simulink model "dynmodelinglinearmpc"  (R2019a)
settings: Solver=FixedStepAuto  StartTime=0.0  StopTime=25  RelTol=1e-3
model workspace (MAT data in the model file):
  op_trim1 : opcond.OperatingReport (value not decoded)
values from neighbouring files (symbols this model uses):
  k = convhulln(p)    [main.m]
undefined symbols (not defined in the file or in its folder): J, L, Mf, R, Rc, Rw
libraries: mpclib x1, mobileRoboticsLib x1
settings Model: Creator=Malicious  LastModifiedBy=colson
settings DataIOCC: ExternalInput=getinputstruct(op_trim1)  InitialState=getstatestruct(op_trim1)  LoadExternalInput=on  ReturnWorkspaceOutputs=off
settings DebuggingCC: PregeneratedLibrarySubsystemCodeDiagnostic=none  ArithmeticOperatorsInVariantConditions=warning
settings SFSimCC: SimUseLocalCustomCode=off
settings RTWCC: RTWUseLocalCustomCode=off

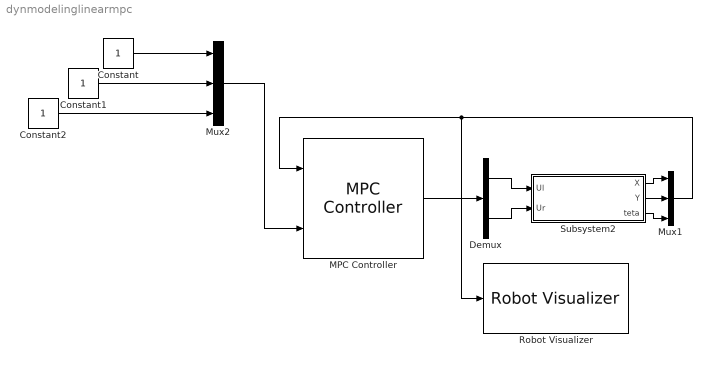
== system dynmodelinglinearmpc ==
  Constant : Constant
  Constant1 : Constant
  Constant2 : Constant
  Demux : Demux  Outputs=2
  MPC Controller : mpclib/MPC Controller  SCDEnableBlockLinearizationSpecification=on  mpcobj=mpc1  is_multiple=0  enable_value=0  return_u0=off  updateMPCinCallerWorkspace=on  md_inport=off  mv_inport=off  uref_inport=off  return_cost=off  return_mvseq=off  return_qpstatus=off  return_xseq=off  return_state=off  return_ovseq=off  state_inport=off  umin_inport=off  umax_inport=off  ymin_inport=off  ymax_inport=off  cc_inport=off  ywt_inport=off  uwt_inport=off  duwt_inport=off  rhoeps_inport=off  pm_inport=off  MaximumP=10  HorizonChoice=FixedHorizon  n_ts=0.1  n_p=10  n_mv=2  n_md=0  n_ud=0  n_mo=3  n_uo=0  BlockDataType=double  SampleTimeInherited=off  switch_inport=off
  Mux1 : Mux  Inputs=3
  Mux2 : Mux  Inputs=3
  Robot Visualizer : mobileRoboticsLib/Environments/Robot Visualizer  robotRadius=0.2  showTrajectory=on  hasWaypoints=off  hasLidar=off  sensorOffset=[ 0, 0 ]  scanAngles=[ -pi/4, 0, pi/4 ]  hasObjDetector=off  objDetectorOffset=[ 0, 0 ]  objDetectorAngle=0  objDetectorFOV=pi/4  objDetectorMaxRange=5  objectColors=[ 1, 0, 0; 0, 1, 0; 0, 0, 1 ]  objectMarkers=s
      settings: SourceProductName=Mobile Robotics Simulation Library
  Subsystem2 : Subsystem
  wires:
  MPC Controller/1 -> Demux/1
  Mux1/1 -> Robot Visualizer/1, MPC Controller/1
  Subsystem2/3(teta) -> Mux1/3
  Subsystem2/2(Y) -> Mux1/2
  Subsystem2/1(X) -> Mux1/1
  Demux/1 -> Subsystem2/1(Ul)
  Demux/2 -> Subsystem2/2(Ur)
  Constant/1 -> Mux2/1
  Constant1/1 -> Mux2/2
  Constant2/1 -> Mux2/3
  Mux2/1 -> MPC Controller/2

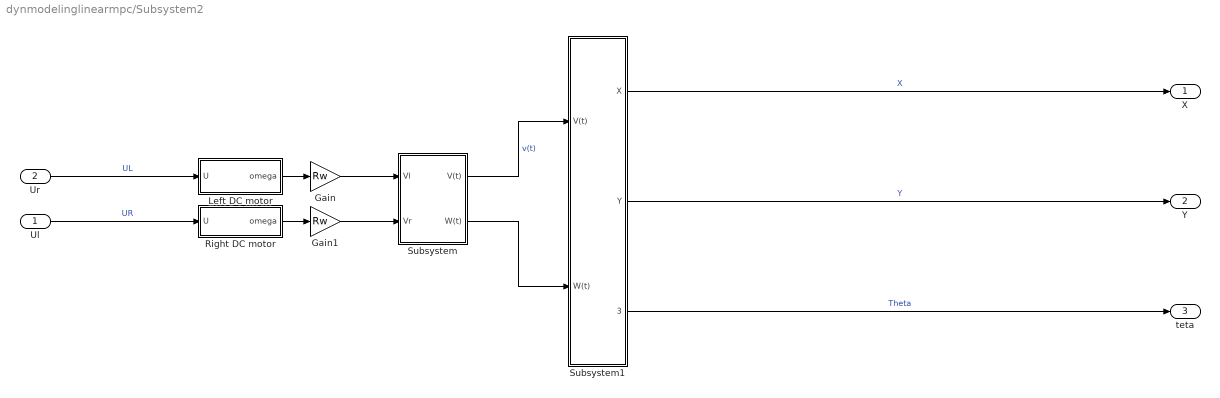
== system dynmodelinglinearmpc/Subsystem2 ==
  Ul : Inport
  Ur : Inport  Port=2
  Gain : Gain  Gain=Rw
  Gain1 : Gain  Gain=Rw
  Left DC motor : Subsystem
  Right DC motor : Subsystem
  Subsystem : Subsystem
  Subsystem1 : Subsystem
  X : Outport
  Y : Outport  Port=2
  teta : Outport  Port=3
  wires:
  Subsystem/1(V(t)) -> Subsystem1/1(V(t))  "v(t)"
  Ur/1 -> Left DC motor/1(U)  "UL"
  Subsystem/2(W(t)) -> Subsystem1/2(W(t))
  Right DC motor/1(omega) -> Gain1/1
  Subsystem1/3(Theta) -> teta/1  "Theta"
  Ul/1 -> Right DC motor/1(U)  "UR"
  Subsystem1/1(X) -> X/1  "X"
  Gain1/1 -> Subsystem/2(Vr)
  Left DC motor/1(omega) -> Gain/1
  Gain/1 -> Subsystem/1(Vl)
  Subsystem1/2(Y) -> Y/1  "Y"

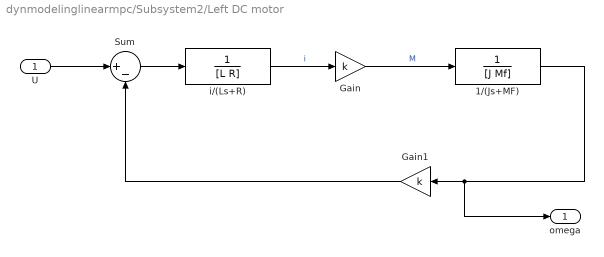
== system dynmodelinglinearmpc/Subsystem2/Left DC motor ==
  U : Inport
  1/(Js+MF) : TransferFcn  Denominator=[J Mf]
  Gain : Gain  Gain=k
  Gain1 : Gain  Gain=k
  Sum : Sum  Inputs=|+-
  i/(Ls+R) : TransferFcn  Denominator=[L R]
  omega : Outport
  wires:
  1/(Js+MF)/1 -> omega/1, Gain1/1
  i/(Ls+R)/1 -> Gain/1  "i"
  Gain1/1 -> Sum/2
  U/1 -> Sum/1
  Sum/1 -> i/(Ls+R)/1
  Gain/1 -> 1/(Js+MF)/1  "M"

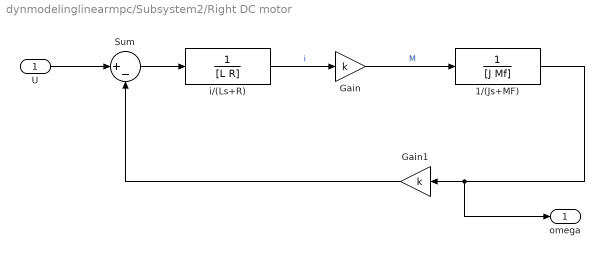
== system dynmodelinglinearmpc/Subsystem2/Right DC motor ==
  U : Inport
  1/(Js+MF) : TransferFcn  Denominator=[J Mf]
  Gain : Gain  Gain=k
  Gain1 : Gain  Gain=k
  Sum : Sum  Inputs=|+-
  i/(Ls+R) : TransferFcn  Denominator=[L R]
  omega : Outport
  wires:
  1/(Js+MF)/1 -> omega/1, Gain1/1
  i/(Ls+R)/1 -> Gain/1  "i"
  Gain1/1 -> Sum/2
  U/1 -> Sum/1
  Sum/1 -> i/(Ls+R)/1
  Gain/1 -> 1/(Js+MF)/1  "M"

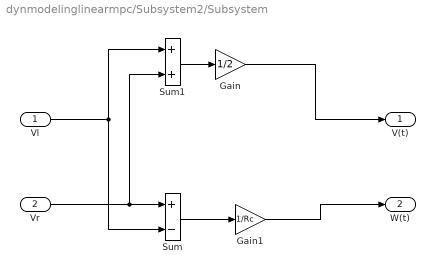
== system dynmodelinglinearmpc/Subsystem2/Subsystem ==
  Vl : Inport
  Vr : Inport  Port=2
  Gain : Gain  Gain=1/2
  Gain1 : Gain  Gain=1/Rc
  Sum : Sum  Inputs=+-
  Sum1 : Sum
  V(t) : Outport
  W(t) : Outport  Port=2
  wires:
  Vr/1 -> Sum/1, Sum1/2
  Vl/1 -> Sum/2, Sum1/1
  Sum1/1 -> Gain/1
  Sum/1 -> Gain1/1
  Gain1/1 -> W(t)/1
  Gain/1 -> V(t)/1

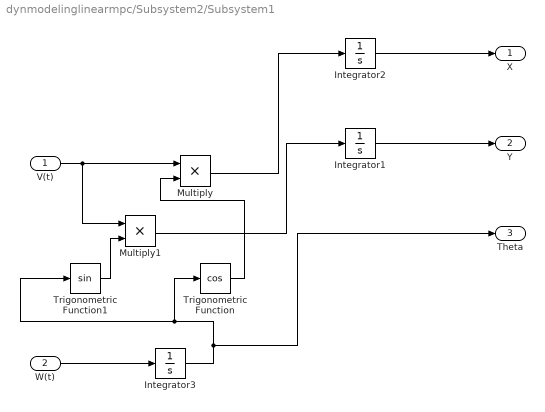
== system dynmodelinglinearmpc/Subsystem2/Subsystem1 ==
  V(t) : Inport
  W(t) : Inport  Port=2
  Integrator1 : Integrator
  Integrator2 : Integrator
  Integrator3 : Integrator
  Multiply : Product
  Multiply1 : Product
  Trigonometric Function : Trigonometry  Operator=cos
  Trigonometric Function1 : Trigonometry
  X : Outport
  Y : Outport  Port=2
  Theta : Outport  Port=3
  wires:
  Integrator3/1 -> Theta/1, Trigonometric Function1/1, Trigonometric Function/1
  Integrator2/1 -> X/1
  Integrator1/1 -> Y/1
  W(t)/1 -> Integrator3/1
  V(t)/1 -> Multiply1/1, Multiply/1
  Trigonometric Function/1 -> Multiply/2
  Multiply/1 -> Integrator2/1
  Trigonometric Function1/1 -> Multiply1/2
  Multiply1/1 -> Integrator1/1
